simulink library "poc_new"  (Simulink 8.1)
settings: Solver=ode1  StartTime=0.0  StopTime=Inf  FixedStep=0.001  RelTol=1e-3
PostLoadFcn:
  | , if any(exist('dsrtsu_mdlpostloadfcn', 'file') == [2, 3, 6]), try dsrtsu_mdlpostloadfcn('Execute', bdroot); catch fprintf('Error in PostLoadFcn (dsrtsu_mdlpostloadfcn) for model "%s":\n %s\n', bdroot, lasterr); end, end,
undefined symbols (not defined in the file or in its folder): KIFO_LongPotentInc_perc, KIFO_PotentDec_perc, KIFO_PotentiallityLimit_num, KIFO_ShortPotentInc_perc, ZERO_FLOAT
libraries: hcu_lib x1, opv x1, simulink x1
settings Model: DSRTSU_INTERNAL_RTI_VER=450  DSRTSU_INTERNAL_RTI_TYPE=rti1401  RTICANMMDATA=struct('GeneralSetupData',struct('modelroot','D:\PROJECTS\HAITEC\TAIWAN_HAITEC_SVN\trunk\AdasDragon\software\sw_development\arch\app\ifo','generalsettings',struct('filesettings',struct('destfolder',struct('Name','RTICANMM_FILES','Check',1),'buildfolder',struct('Name','.','Check',1),'AbsDestfolder',struct('Name','D:\PROJECTS\HAITEC\TAIWAN_HAITEC_SVN\trunk\AdasDragon\software\sw_development\arch\app\ifo\RTICANMM_FILES'),'AbsBuildfolder',struct('Name','D:\PROJECTS\HAITEC\TAIWAN_HAITEC_SVN\trunk\AdasDragon\software\sw_development\arch\app\ifo'))),'options',struct('addpaths',1,'rmpaths',1,'addtrcexclusion',logical(1),'cannavigator',struct('checkmonitoring',0),'show_usrtrc',0,'use_usrtrc',0),'advanced',struct('options',[1 1 1 1 1 1 1 1 1 1 1 1 1 1 1 1 1 1 1 1 1 1 1 1 1 1 1 1 1 1 1 1 1 1 1 1 1 1 1 1 1 1 1 1 1 1 1 1 1 1 1 1 1 1 1 1 1 1 1 1 1 1 1 1 1 1 1 1 1 1 1 1 1 1 1 1 1 1 1 1 1 1 1 1 1 1 1 1 1 1 1 1 1 1 1 1 1 1 1 1]),'MPSetup',{{}},'modelname','poc','block','poc'))  DSRTSU_INTERNAL_RTIFPGA=40  Creator=tescamilla  LastModifiedBy=tescamilla

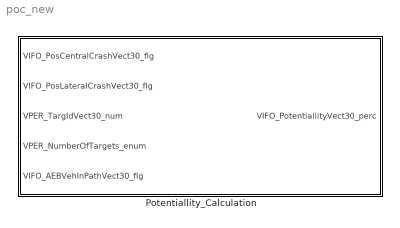
== system poc_new ==
  Potentiallity_Calculation : Subsystem

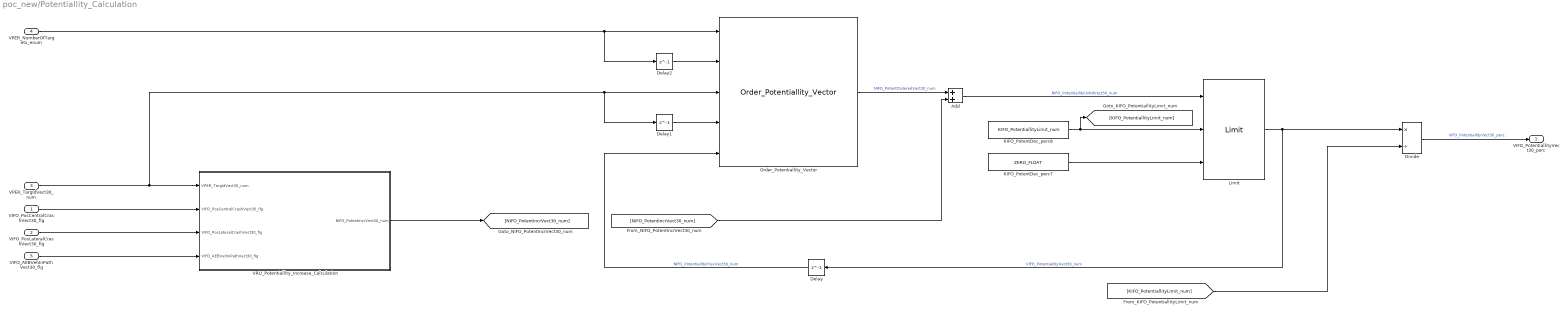
== system poc_new/Potentiallity_Calculation ==
  VIFO_PosCentralCrashVect30_flg : Inport
  VIFO_PosLateralCrashVect30_flg : Inport  Port=2
  VPER_TargIdVect30_num : Inport  Port=3
  VPER_NumberOfTargets_enum : Inport  Port=4
  VIFO_AEBVehInPathVect30_flg : Inport  Port=5
  Add : Sum
  Delay : Delay  DelayLength=1  InitialCondition=zeros(1,30)
  Delay1 : Delay  DelayLength=1  InitialCondition=0
  Delay2 : Delay  DelayLength=1  InitialCondition=0
  Divide : Product  Inputs=*/
  KIFO_PotentDec_perc7 : Constant  Value=ZERO_FLOAT
  KIFO_PotentDec_perc8 : Constant  Value=KIFO_PotentiallityLimit_num
  Limit : hcu_lib/Limit  SystemSampleTime=-1
  Order_Potentiallity_Vector : opv/Order_Potentiallity_Vector
  VRU_Potentiallity_Increase_Calculation : Subsystem
  VIFO_PotentiallityVect30_perc : Outport
  wires:
  KIFO_PotentDec_perc7/1 -> Limit/3
  Add/1 -> Limit/1  "NIFO_PotentiallityUnltdVect30_num"
  KIFO_PotentDec_perc8/1 -> [KIFO_PotentiallityLimit_num], Limit/2
  Delay/1 -> Order_Potentiallity_Vector/5  "NIFO_PotentiallityPrevVect30_num"
  [KIFO_PotentiallityLimit_num] -> Divide/2
  Divide/1 -> VIFO_PotentiallityVect30_perc/1  "VIFO_PotentiallityVect30_perc"
  VPER_TargIdVect30_num/1 -> VRU_Potentiallity_Increase_Calculation/1(VPER_TargIdVect30_num), Order_Potentiallity_Vector/3, Delay1/1
  Limit/1 -> Delay/1, Divide/1  "VIFO_PotentiallityVect30_num"
  VPER_NumberOfTargets_enum/1 -> Order_Potentiallity_Vector/1, Delay2/1
  Order_Potentiallity_Vector/1 -> Add/1  "NIFO_PotentOrderedVect30_num"
  [NIFO_PotentIncrVect30_num] -> Add/2
  VIFO_PosCentralCrashVect30_flg/1 -> VRU_Potentiallity_Increase_Calculation/2(VIFO_PosCentralCrashVect30_flg)
  VIFO_PosLateralCrashVect30_flg/1 -> VRU_Potentiallity_Increase_Calculation/3(VIFO_PosLateralCrashVect30_flg)
  VRU_Potentiallity_Increase_Calculation/1(NIFO_PotentIncrVect30_num) -> [NIFO_PotentIncrVect30_num]
  Delay1/1 -> Order_Potentiallity_Vector/4
  Delay2/1 -> Order_Potentiallity_Vector/2
  VIFO_AEBVehInPathVect30_flg/1 -> VRU_Potentiallity_Increase_Calculation/4(VIFO_AEBVehInPathVect30_flg)

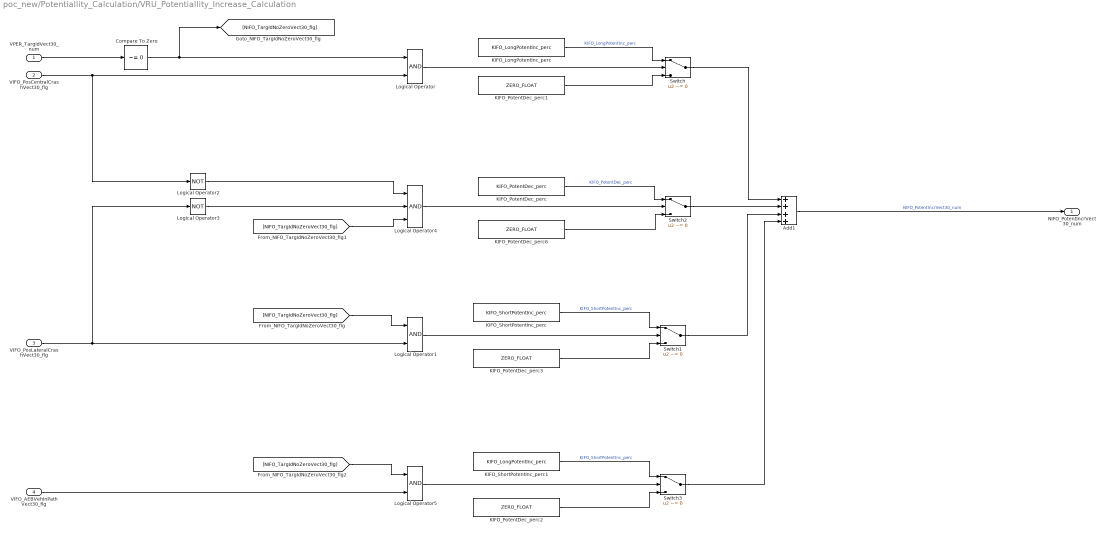
== system poc_new/Potentiallity_Calculation/VRU_Potentiallity_Increase_Calculation ==
  VPER_TargIdVect30_num : Inport
  VIFO_PosCentralCrashVect30_flg : Inport  Port=2
  VIFO_PosLateralCrashVect30_flg : Inport  Port=3
  VIFO_AEBVehInPathVect30_flg : Inport  Port=4
  Add1 : Sum  Inputs=++++
  Compare To Zero : simulink/Logic and Bit Operations/Compare To Zero  relop=~=  OutDataTypeStr=boolean
  KIFO_LongPotentInc_perc : Constant  Value=KIFO_LongPotentInc_perc
  KIFO_PotentDec_perc : Constant  Value=KIFO_PotentDec_perc
  KIFO_PotentDec_perc{1..3,6} (4 alike) : Constant  Value=ZERO_FLOAT
  KIFO_ShortPotentInc_perc : Constant  Value=KIFO_ShortPotentInc_perc
  KIFO_ShortPotentInc_perc1 : Constant  Value=KIFO_LongPotentInc_perc
  Logical Operator : Logic  AllPortsSameDT=off  OutDataTypeStr=boolean
  Logical Operator1 : Logic  AllPortsSameDT=off  OutDataTypeStr=boolean
  Logical Operator2 : Logic  Operator=NOT  AllPortsSameDT=off  OutDataTypeStr=boolean
  Logical Operator3 : Logic  Operator=NOT  AllPortsSameDT=off  OutDataTypeStr=boolean
  Logical Operator4 : Logic  Inputs=3  AllPortsSameDT=off  OutDataTypeStr=boolean
  Logical Operator5 : Logic  AllPortsSameDT=off  OutDataTypeStr=boolean
  Switch{,1..3} (4 alike) : Switch  Criteria=u2 ~= 0
  NIFO_PotentIncrVect30_num : Outport
  wires:
  VPER_TargIdVect30_num/1 -> Compare To Zero/1
  Logical Operator4/1 -> Switch2/2
  Logical Operator/1 -> Switch/2
  VIFO_PosCentralCrashVect30_flg/1 -> Logical Operator/2, Logical Operator2/1
  VIFO_PosLateralCrashVect30_flg/1 -> Logical Operator1/2, Logical Operator3/1
  KIFO_PotentDec_perc1/1 -> Switch/3
  Compare To Zero/1 -> Logical Operator/1, [NIFO_TargIdNoZeroVect30_flg]
  [NIFO_TargIdNoZeroVect30_flg] -> Logical Operator1/1
  Add1/1 -> NIFO_PotentIncrVect30_num/1  "NIFO_PotentIncrVect30_num"
  Logical Operator2/1 -> Logical Operator4/1
  Switch2/1 -> Add1/2
  Switch/1 -> Add1/1
  [NIFO_TargIdNoZeroVect30_flg] -> Logical Operator4/3
  KIFO_ShortPotentInc_perc/1 -> Switch1/1  "KIFO_ShortPotentInc_perc"
  KIFO_PotentDec_perc3/1 -> Switch1/3
  Logical Operator3/1 -> Logical Operator4/2
  Switch1/1 -> Add1/3
  KIFO_LongPotentInc_perc/1 -> Switch/1  "KIFO_LongPotentInc_perc"
  KIFO_PotentDec_perc/1 -> Switch2/1  "KIFO_PotentDec_perc"
  KIFO_PotentDec_perc6/1 -> Switch2/3
  Logical Operator1/1 -> Switch1/2
  VIFO_AEBVehInPathVect30_flg/1 -> Logical Operator5/2
  [NIFO_TargIdNoZeroVect30_flg] -> Logical Operator5/1
  KIFO_ShortPotentInc_perc1/1 -> Switch3/1  "KIFO_ShortPotentInc_perc"
  KIFO_PotentDec_perc2/1 -> Switch3/3
  Switch3/1 -> Add1/4
  Logical Operator5/1 -> Switch3/2
